simulink model "pfa1008"  (R2025a)
settings: Solver=VariableStepAuto  StartTime=0.0  StopTime=1e-4  RelTol=1e-3
InitFcn:
  | coeffs;
undefined symbols (not defined in the file or in its folder): S, vsva2197, xcvc1902
libraries: aieBasic x20, aieUtilities x5, dspsrcs4 x4, hlsBasic x2, vmcUtilities x1
(part 1 of 2)
settings Model: Creator=robg  LastModifiedBy=sdegala
settings RTWCC: GPUComputeCapability=3.5

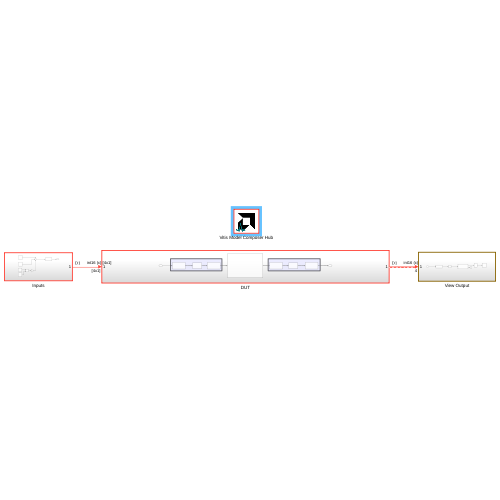
[thumbnail: Simulink's stored preview of the top-level diagram]
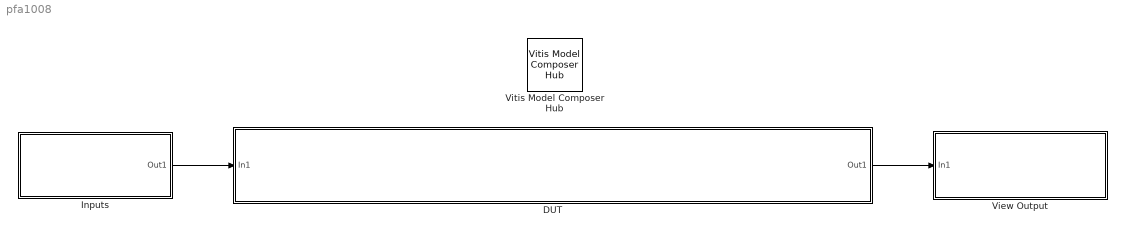
== system pfa1008 ==
  DUT : Subsystem
  Inputs : Subsystem
  View Output : Subsystem
  Vitis Model Composer Hub : vmcUtilities/Vitis Model Composer Hub  Tag=genX  CodeGeneration=off  SubsystemName=DUT  DUTSubsystemName=pfa1008  BlockHierPath=pfa1008/DUT  CompilationType=VitisCompilation  SubsystemType=DUTNode  ExportTypeV2=Graph Code  AIEArrayConfig=Use entire AIE array  StartColumn=1  NumberOfColumns=1  TargetDirectory=./code  exportDesign=on  analyzeDesign=off  validateDesignOnHw=off  ExportType=Vitis Subsystem  IpVendor=xilinx.com  IpLibrary=hls  IpName=pfa1008_permute_o_wrapper  IpVersion=1.0  IpHWLanguage=Verilog  AieCompilerOptions={}  AieSimulatorOptions={''}  CreateTestbench=off  TestbenchStackSize=10  RunRtlSim=off  RunCSim=off  RunAieSim=on  AieSimTimeout=50000  RunAieSimProfiling=off  LaunchVitisAnalyzer=off  PlotOutput=off  RunX86Sim=off  X86SimTimeout=10  GenHwImage=off  GenLibadfXo=on  GenHwValidationCode=on  PlatformType=Specify Platform  Platform=/proj/xbuilds/SWIP/9999.0_0818_1732/installs/lin64/2025.2/Vitis/base_platforms/xilinx_vck190_base_202520_1/xilinx_vck190_base_202520_1.xpfm  HwSystemType=Baremetal  HwValidationTarget=hw_emu  ProjDevice=Versal VCK190 Evaluation Platform (xcvc1902-vsva2197-2MP-e-S)  ProjDevicePart=xcvc1902-vsva2197-2MP-e-S  AIEType=AIE  SamplePeriod=-1  ClockFrequency=200  DataPathParallelism=1  xilinxfamily=versalaicore  part=xcvc1902  speed=-2MP-e-S  package=vsva2197  directory=./netlist  testbench=off  incr_netlist=off  synthesis_tool=Vivado  clock_wrapper=Clock Enables  dbl_ovrd=According to Block Masks  dcm_input_clock_period=10  sysclk_period=10  simulink_period=1  eval_field=0  IPInfoJsonString="{\"DUTSubsystemName\":\"DUT\",\"HLSKernel\":[{\"SubsystemName\":\"pfa1008_permute_i_wrapper\",\"FpgaClockFreq\":\"200\",\"IPName\":\"pfa1008_permute_i_wrapper\",\"IPLibrary\":\"hls\",\"TargetDirectory\":\"./code\",\"FreqHz\":\"200000000\",\"KernelFunction\":\"pfa1008_permute_i_wrapper\"},{\"SubsystemName\":\"pfa1008_permute_o_wrapper\",\"FpgaClockFreq\":\"200\",\"IPName\":\"pfa1008_permute_o_wrapper\",\"IPLibrary\":\"hls\",\"TargetDirectory\":\"./code\",\"FreqHz\":\"200000000\",\"KernelFunction\":\"pfa1008_permute_o_wrapper\"}],\"SubsystemTag\":\"DUTNode\",\"AIESubsystem\":{\"SubsystemName\":\"pfa1008_aie\",\"TargetDirectory\":\"./code\",\"AIEArrayConfig\":\"Use entire AIE array\",\"StartColumn\":\"1\",\"NumberOfColumns\":\"1\"}}"  LogFileName=/proj/xhdhdstaff5/sdegala/Head1/HEAD/VMC_2025_2_July/Examples/AIENGINE_plus_PL/AIE_HLS/Prime_Factor_FFT/code/model_composer.log  NThreads=4  IPConfigFile=/tmp/vmctmp-6835010160091439353/pfa1008_ipconfig.json
  wires:
  Inputs/1(Out1) -> DUT/1(In1)
  DUT/1(Out1) -> View Output/1(In1)

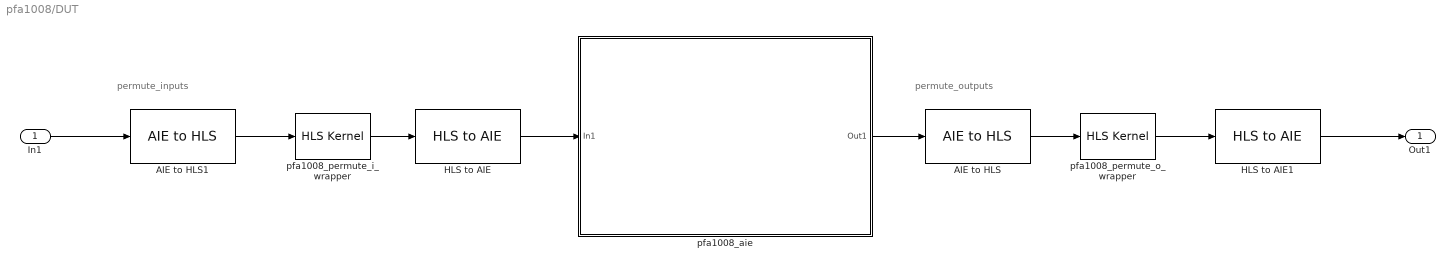
== system pfa1008/DUT ==
  note: permute_outputs
  note: permute_inputs
  In1 : Inport
  AIE to HLS : aieUtilities/AIE to HLS  OutputType=ufix128  OutputSize=252  AllowMultiRate=off  InputType=int8
  AIE to HLS1 : aieUtilities/AIE to HLS  OutputType=ufix128  OutputSize=1  AllowMultiRate=off  InputType=int8
  HLS to AIE : aieUtilities/HLS to AIE  OutputType=cint16  OutputSize=1008  AllowMultiRate=off  InputType=cint16
  HLS to AIE1 : aieUtilities/HLS to AIE  OutputType=cint16  OutputSize=4  AllowMultiRate=off  InputType=cint16
  pfa1008_aie : Subsystem
  pfa1008_permute_i_wrapper : hlsBasic/HLS Kernel  PortNames={'return'; 'sig_i'; 'sig_o'}  PortSerializedTypes={'{Bv}'; '{R{Thls::stream{2{t{Tap_uint{1{t{}128}}}}{t{}0}}}}'; '{R{Thls::stream{2{t{Tap_uint{1{t{}128}}}}{t{}0}}}}'}  FunctionTemplateSpecKind=none  FunctionTemplateParamNames={}  FunctionTemplateParamKinds={}  FunctionTemplateParamTypes={}  FunctionTemplateParamValues={}  PortSynchronicities={'auto'; 'auto'}  PortSignalSizes={0.000000000000000000e+00; 2.520000000000000000e+02}  PortParameterValues={}  PortAttributesTable={ 'Input', 'sig_i', 'hls::stream< ap_uint< 128 >, 0 > &', '', ''; 'Output', 'sig_o', 'hls::stream< ap_uint< 128 >, 0 > &', '', '252' }  PortAttributesEnablement={'off', 'off', 'off', 'off', 'off';'off', 'off', 'off', 'off', 'on'}  PortParametersTable={}  SampleTime=-1  PortDirectionTable={ 'sig_i', 'hls::stream< ap_uint< 128 >, 0 > &', 'Input', 'Port'; 'sig_o', 'hls::stream< ap_uint< 128 >, 0 > &', 'Output', 'Port' }  FunctionTemplateParams={}  FunctionTemplateParamsEnables={}  FunctionTemplateParamsVisible=off  FunctionDeclTypeOptions=C[1 1]@t7@<empty>  PortDirectionTabVisible=on  ArgDirections={1.000000000000000000e+00; 2.000000000000000000e+00}  ArgInterfaceTypes={1.000000000000000000e+00; 1.000000000000000000e+00}  FunctionIndex=1  FormalArgDecls={'hls::stream< ap_uint< 128 >, 0 > & sig_i', 'hls::stream< ap_uint< 128 >, 0 > & sig_o'}  SimLibPath=''  FunctionTabVisible=on  FunctionDescription=void pfa1008_permute_i_wrapper(hls::stream< ap_uint< 128 >, 0 > & sig_i, hls::stream< ap_uint< 128 >, 0 > & sig_o)  blockJsonConstraints=[]  deprecateConstraints=0  KernelHeaderFile=./hls/pfa1008_permute_i/pfa1008_permute_i.h  KernelFunction=pfa1008_permute_i_wrapper  KernelFunctionSelect=<empty>  KernelSourceFile=./hls/pfa1008_permute_i/pfa1008_permute_i.cpp  KernelSearchPaths={}  PreProcOptions={}
  pfa1008_permute_o_wrapper : hlsBasic/HLS Kernel  PortNames={'return'; 'sig_i'; 'sig_o'}  PortSerializedTypes={'{Bv}'; '{R{Thls::stream{2{t{Tap_uint{1{t{}128}}}}{t{}0}}}}'; '{R{Thls::stream{2{t{Tap_uint{1{t{}128}}}}{t{}0}}}}'}  FunctionTemplateSpecKind=none  FunctionTemplateParamNames={}  FunctionTemplateParamKinds={}  FunctionTemplateParamTypes={}  FunctionTemplateParamValues={}  PortSynchronicities={'auto'; 'auto'}  PortSignalSizes={0.000000000000000000e+00; 1.000000000000000000e+00}  PortParameterValues={}  PortAttributesTable={ 'Input', 'sig_i', 'hls::stream< ap_uint< 128 >, 0 > &', '', ''; 'Output', 'sig_o', 'hls::stream< ap_uint< 128 >, 0 > &', '', '1' }  PortAttributesEnablement={'off', 'off', 'off', 'off', 'off';'off', 'off', 'off', 'off', 'on'}  PortParametersTable={}  SampleTime=-1  PortDirectionTable={ 'sig_i', 'hls::stream< ap_uint< 128 >, 0 > &', 'Input', 'Port'; 'sig_o', 'hls::stream< ap_uint< 128 >, 0 > &', 'Output', 'Port' }  FunctionTemplateParams={}  FunctionTemplateParamsEnables={}  FunctionTemplateParamsVisible=off  FunctionDeclTypeOptions=C[1 1]@t7@<empty>  PortDirectionTabVisible=on  ArgDirections={1.000000000000000000e+00; 2.000000000000000000e+00}  ArgInterfaceTypes={1.000000000000000000e+00; 1.000000000000000000e+00}  FunctionIndex=1  FormalArgDecls={'hls::stream< ap_uint< 128 >, 0 > & sig_i', 'hls::stream< ap_uint< 128 >, 0 > & sig_o'}  SimLibPath=''  FunctionTabVisible=on  FunctionDescription=void pfa1008_permute_o_wrapper(hls::stream< ap_uint< 128 >, 0 > & sig_i, hls::stream< ap_uint< 128 >, 0 > & sig_o)  blockJsonConstraints=[]  deprecateConstraints=0  KernelHeaderFile=./hls/pfa1008_permute_o/pfa1008_permute_o.h  KernelFunction=pfa1008_permute_o_wrapper  KernelFunctionSelect=<empty>  KernelSourceFile=./hls/pfa1008_permute_o/pfa1008_permute_o.cpp  KernelSearchPaths={}  PreProcOptions={}
  Out1 : Outport
  wires:
  HLS to AIE/1 -> pfa1008_aie/1(In1)
  HLS to AIE1/1 -> Out1/1
  In1/1 -> AIE to HLS1/1
  AIE to HLS1/1 -> pfa1008_permute_i_wrapper/1
  pfa1008_permute_i_wrapper/1 -> HLS to AIE/1
  pfa1008_aie/1(Out1) -> AIE to HLS/1
  pfa1008_permute_o_wrapper/1 -> HLS to AIE1/1
  AIE to HLS/1 -> pfa1008_permute_o_wrapper/1

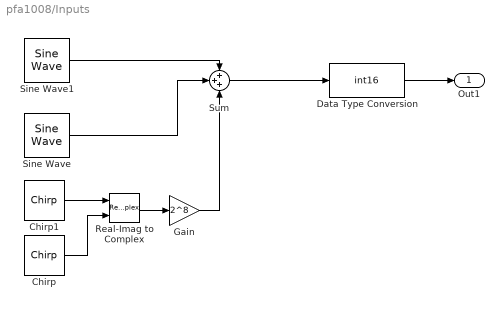
== system pfa1008/Inputs ==
  Chirp : dspsrcs4/Chirp  sweep=Linear  mode=Unidirectional  f0=100/1008*(1e9)  f1=200/1008*(1e9)  t1=4032*(1e-9)  Tsweep=4032*(1e-9)  phase=0  Ts=1e-9  spf=4  datatype=double  OutputFrames=off
  Chirp1 : dspsrcs4/Chirp  sweep=Linear  mode=Unidirectional  f0=100/1008*(1e9)  f1=200/1008*(1e9)  t1=4032*(1e-9)  Tsweep=4032*(1e-9)  phase=pi/2  Ts=1e-9  spf=4  datatype=double  OutputFrames=off
  Data Type Conversion : DataTypeConversion  OutDataTypeStr=int16  SaturateOnIntegerOverflow=off  RndMeth=Floor
  Gain : Gain  Gain=2^8  OutDataTypeStr=double
  Real-Imag to Complex : RealImagToComplex
  Sine Wave : dspsrcs4/Sine Wave  Amplitude=2^8  Frequency=128/1008*(1e9)  Phase=0  SampleMode=Discrete  OutComplex=Complex  CompMethod=Trigonometric fcn  TableSize=Speed  SampleTime=1e-9  SamplesPerFrame=4  ResetState=Restart at time zero  OutputFrames=off  dataType=double  wordLen=16  udDataType=sfix(16)  fracBitsMode=Best precision  numFracBits=15  OutDataTypeStr=double  LastOutDataTypeStr=double
  Sine Wave1 : dspsrcs4/Sine Wave  Amplitude=2^8  Frequency=400/1008*(1e9)  Phase=0  SampleMode=Discrete  OutComplex=Complex  CompMethod=Trigonometric fcn  TableSize=Speed  SampleTime=1e-9  SamplesPerFrame=4  ResetState=Restart at time zero  OutputFrames=off  dataType=double  wordLen=16  udDataType=sfix(16)  fracBitsMode=Best precision  numFracBits=15  OutDataTypeStr=double  LastOutDataTypeStr=double
  Sum : Sum  Inputs=+++
  Out1 : Outport
  wires:
  Sine Wave1/1 -> Sum/1
  Sine Wave/1 -> Sum/2
  Sum/1 -> Data Type Conversion/1
  Data Type Conversion/1 -> Out1/1
  Gain/1 -> Sum/3
  Real-Imag to Complex/1 -> Gain/1
  Chirp/1 -> Real-Imag to Complex/2
  Chirp1/1 -> Real-Imag to Complex/1

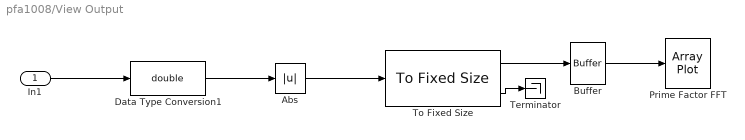
== system pfa1008/View Output ==
  In1 : Inport
  Abs : Abs  OutDataTypeStr=double  SaturateOnIntegerOverflow=off
  Buffer : Buffer  N=1008  OutputFrames=off
  Data Type Conversion1 : DataTypeConversion  OutDataTypeStr=double  SaturateOnIntegerOverflow=off  RndMeth=Floor
  Prime Factor FFT : ArrayPlot  WindowPosition=[1116.000000,386.000000,800.000000,500.000000,]  Visible=on  ScopeFrameLocation=window  MaximizeAxes=Off  YLimits=[-4095.8765 36862.8885]
  Terminator : Terminator
  To Fixed Size : aieUtilities/To Fixed Size  Mode=Produce a valid output signal  OutputSize=Inherit: Same as input  CopyMethod=Buffer samples to form output  HasStatusOutput=on
  wires:
  Abs/1 -> To Fixed Size/1
  Data Type Conversion1/1 -> Abs/1
  To Fixed Size/2 -> Terminator/1
  Buffer/1 -> Prime Factor FFT/1
  To Fixed Size/1 -> Buffer/1
  In1/1 -> Data Type Conversion1/1

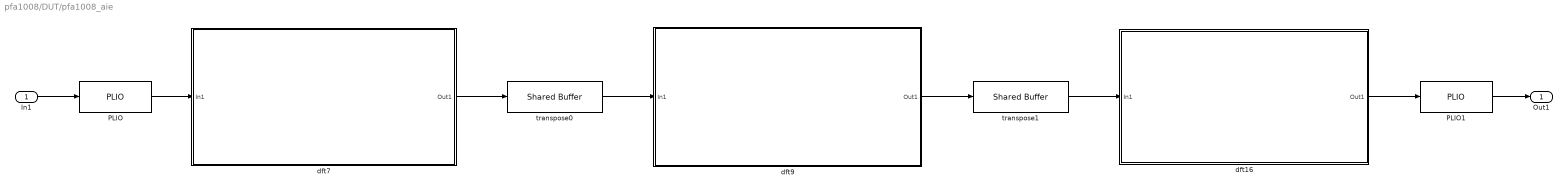
== system pfa1008/DUT/pfa1008_aie ==
  In1 : Inport
  PLIO : aieBasic/PLIO  PlioWidth=64  PlioFreqSpec=on  PlioFreq=625  ColLocation=0  channel=0  blockJsonConstraints=[]  deprecateConstraints=0
  PLIO1 : aieBasic/PLIO  PlioWidth=64  PlioFreqSpec=on  PlioFreq=625  ColLocation=0  channel=0  blockJsonConstraints=[]  deprecateConstraints=0
  dft16 : Subsystem
  dft7 : Subsystem
  dft9 : Subsystem
  transpose0 : aieBasic/Shared Buffer  DataType=cint16  NumBuffer=2  BufferDim=[8,16,16]  NumInput=1  NumOutput=1  RepetitionCount=0  Input0Tiling=struct('buffer_dimension', [8,16,16], 'tiling_dimension', [1,1,1], 'offset', [0,0,0], 'tile_traversal', [struct('dimension', 0, 'stride', 1, 'wrap', 7) struct('dimension', 1, 'stride', 1, 'wrap', 9) struct('dimension', 2, 'stride', 1, 'wrap', 16)])  Input1Tiling=[]  Input2Tiling=[]  Input3Tiling=[]  Input4Tiling=[]  Input5Tiling=[]  Output0Tiling=struct('buffer_dimension', [8,16,16], 'tiling_dimension', [1,1,1], 'offset', [0,0,0], 'tile_traversal', [struct('dimension', 1, 'stride', 1, 'wrap', 9) struct('dimension', 2, 'stride', 1, 'wrap', 16) struct('dimension', 0, 'stride', 1, 'wrap', 7)])  Output1Tiling=[]  Output2Tiling=[]  Output3Tiling=[]  Output4Tiling=[]  Output5Tiling=[]  InBuffDims={8, 16, 16}  InTilingDims={1, 1, 1}  InOffsets={0, 0, 0}  InTileTraveseDims={0,1,2}  InTileTraveseStrides={1,1,1}  InTileTraveseWraps={7,9,16}  InPacketPortIDs={}  InRepetitions={}  InBoundaryDims={}  OutBuffDims={8, 16, 16}  OutTilingDims={1, 1, 1}  OutOffsets={0, 0, 0}  OutTileTraveseDims={1,2,0}  OutTileTraveseStrides={1,1,1}  OutTileTraveseWraps={9,16,7}  OutPacketPortIDs={}  OutRepetitions={}  OutBoundaryDims={}  BufferDimStr={8, 16, 16}  blockJsonConstraints=[]  deprecateConstraints=0
  transpose1 : aieBasic/Shared Buffer  DataType=cint16  NumBuffer=2  BufferDim=[8,16,16]  NumInput=1  NumOutput=1  RepetitionCount=0  Input0Tiling=struct('buffer_dimension', [8,16,16], 'tiling_dimension', [1,1,1], 'offset', [0,0,0], 'tile_traversal', [struct('dimension', 1, 'stride', 1, 'wrap', 9) struct('dimension', 2, 'stride', 1, 'wrap', 16) struct('dimension', 0, 'stride', 1, 'wrap', 7)])  Input1Tiling=[]  Input2Tiling=[]  Input3Tiling=[]  Input4Tiling=[]  Input5Tiling=[]  Output0Tiling=struct('buffer_dimension', [8,16,16], 'tiling_dimension', [1,1,1], 'offset', [0,0,0], 'tile_traversal', [struct('dimension', 2, 'stride', 1, 'wrap', 16) struct('dimension', 1, 'stride', 1, 'wrap', 9) struct('dimension', 0, 'stride', 1, 'wrap', 7)])  Output1Tiling=[]  Output2Tiling=[]  Output3Tiling=[]  Output4Tiling=[]  Output5Tiling=[]  InBuffDims={8, 16, 16}  InTilingDims={1, 1, 1}  InOffsets={0, 0, 0}  InTileTraveseDims={1,2,0}  InTileTraveseStrides={1,1,1}  InTileTraveseWraps={9,16,7}  InPacketPortIDs={}  InRepetitions={}  InBoundaryDims={}  OutBuffDims={8, 16, 16}  OutTilingDims={1, 1, 1}  OutOffsets={0, 0, 0}  OutTileTraveseDims={2,1,0}  OutTileTraveseStrides={1,1,1}  OutTileTraveseWraps={16,9,7}  OutPacketPortIDs={}  OutRepetitions={}  OutBoundaryDims={}  BufferDimStr={8, 16, 16}  blockJsonConstraints=[]  deprecateConstraints=0
  Out1 : Outport
  wires:
  PLIO1/1 -> Out1/1
  In1/1 -> PLIO/1
  PLIO/1 -> dft7/1(In1)
  dft7/1(Out1) -> transpose0/1
  transpose0/1 -> dft9/1(In1)
  dft9/1(Out1) -> transpose1/1
  transpose1/1 -> dft16/1(In1)
  dft16/1(Out1) -> PLIO1/1

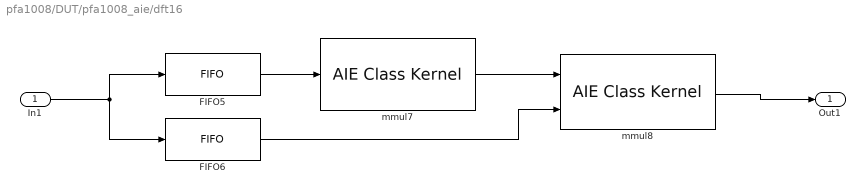
== system pfa1008/DUT/pfa1008_aie/dft16 ==
  In1 : Inport
  FIFO5 : aieBasic/FIFO  FifoDepth=32  FIFOType=0  TileType=0  RowLocation=0  ColLocation=0  channel=0  blockJsonConstraints=[]  deprecateConstraints=0
  FIFO6 : aieBasic/FIFO  FifoDepth=32  FIFOType=0  TileType=0  RowLocation=0  ColLocation=0  channel=0  blockJsonConstraints=[]  deprecateConstraints=0
  mmul7 : aieBasic/AIE Class Kernel  KernelAllAttrs=|  PortNames={'sig_i'; 'acc_o'}  PortSerializedTypes={'{Q2{R{Tadf::input_buffer{2{t{Scint16}}{t{Tadf::extents{1{t{}1008}}}}}}}}'; '{Q2{P{Toutput_cascade{2{t{Scacc64}}{t{Bv}}}}}}'}  PortWindowSizes={1.008000000000000000e+03; 0.000000000000000000e+00}  PortWindowMargins={0.000000000000000000e+00; 0.000000000000000000e+00}  PortSynchronicities={'sync', 'auto'}  PortSignalSizes={0.000000000000000000e+00; 1.008000000000000000e+03}  ClassTemplateSpecKind=none  ClassTemplateParamNames={}  ClassTemplateParamKinds={}  ClassTemplateParamTypes={}  ClassTemplateParamValues={}  ClassCtorParamNames={'coeff_i'}  ClassCtorParamSerializedTypes={'{R{C{Scint16}256}}'}  ClassCtorParamValues={'[32767;32767;32767;32767;32767;32767;32767;32767;32767;30274-12540i;23170-23170i;12540-30274i;0-32768i;-12540-30274i;-23170-23170i;-30274-12540i;32767;23170-23170i;0-32768i;-23170-23170i;-32768;-23170+23170i;0+32767i;23170+23170i;32767;12540-30274i;-23170-23170i;-30274+12540i;0+32767i;30274+12540i;23170-23170i;-12540-30274i;32767;0-32768i;-32768;0+32767i;32767;0-32768i;-32768;0+32767i;32767;-12540-30274i;-23170+23170i;30274+12540i;0-32768i;-30274+12540i;23170+23170i;12540-30274i;32767;-23170-23170i;0+32767i;23170-23170i;-32768;23170+23170i;0-32768i;-23170+23170i;32767;-30274-12540i;23170+23170i;-12540-30274i;0+32767i;12540-30274i;-23170+23170i;30274-12540i;32767;-32768;32767;-32768;32767;-32768;32767;-32768;32767;-30274+12540i;23170-23170i;-12540+30274i;0-32768i;12540+30274i;-23170-23170i;30274+12540i;32767;-23170+23170i;0-32768i;23170+23170i;-32768;23170-23170i;0+32767i;-23170-23170i;32767;-12540+30274i;-23170-23170i;30274-12540i;0+32767i;-30274-12540i;23170-23170i;12540+30274i;32767;0+32767i;-32768;0-32768i;32767;0+32767i;-32768;0-32768i;32767;12540+30274i;-23170+23170i;-30274-12540i;0-32768i;30274-12540i;23170+23170i;-12540+30274i;32767;23170+23170i;0+32767i;-23170+23170i;-32768;-23170-23170i;0-32768i;23170-23170i;32767;30274+12540i;23170+23170i;12540+30274i;0+32767i;-12540+30274i;-23170+23170i;-30274+12540i;32767;32767;32767;32767;32767;32767;32767;32767;-32768;-30274+12540i;-23170+23170i;-12540+30274i;0+32767i;12540+30274i;23170+23170i;30274+12540i;32767;23170-23170i;0-32768i;-23170-23170i;-32768;-23170+23170i;0+32767i;23170+23170i;-32768;-12540+30274i;23170+23170i;30274-12540i;0-32768i;-30274-12540i;-23170+23170i;12540+30274i;32767;0-32768i;-32768;0+32767i;32767;0-32768i;-32768;0+32767i;-32768;12540+30274i;23170-23170i;-30274-12540i;0+32767i;30274-12540i;-23170-23170i;-12540+30274i;32767;-23170-23170i;0+32767i;23170-23170i;-32768;23170+23170i;0-32768i;-23170+23170i;-32768;30274+12540i;-23170-23170i;12540+30274i;0-32768i;-12540+30274i;23170-23170i;-30274+12540i;32767;-32768;32767;-32768;32767;-32768;32767;-32768;-32768;30274-12540i;-23170+23170i;12540-30274i;0+32767i;-12540-30274i;23170+23170i;-30274-12540i;32767;-23170+23170i;0-32768i;23170+23170i;-32768;23170-23170i;0+32767i;-23170-23170i;-32768;12540-30274i;23170+23170i;-30274+12540i;0-32768i;30274+12540i;-23170+23170i;-12540-30274i;32767;0+32767i;-32768;0-32768i;32767;0+32767i;-32768;0-32768i;-32768;-12540-30274i;23170-23170i;30274+12540i;0+32767i;-30274+12540i;-23170-23170i;12540-30274i;32767;23170+23170i;0+32767i;-23170+23170i;-32768;-23170-23170i;0-32768i;23170-23170i;-32768;-30274-12540i;-23170-23170i;-12540-30274i;0-32768i;12540-30274i;23170-23170i;30274-12540i]'}  ClassIndex=1  ClassCtorIndex=1  ClassTabVisible=on  ClassTemplateParamsVisible=off  ClassCtorDeclVisible=on  ClassCtorParamsVisible=on  FunctionTabVisible=on  FunctionDecl=|  PortAttrs={ 'input', 'sig_i', 'adf::input_buffer< cint16, adf::extents< 1008 > > & restrict', '1008', '0', 'sync', ''; 'output', 'acc_o', 'output_cascade< cacc64, void > * restrict', '', '', '', '1008' }  PortAttrsEnables={'off', 'off', 'off', 'off', 'off', 'off', 'off';'off', 'off', 'off', 'off', 'off', 'off', 'on'}  SampleTime=-1  ClassDeclTypeOptions=C[1 1]@t14@class dft16_0;  ClassDecl=class dft16_0;  ClassTemplateParams={}  ClassTemplateParamsEnables={}  ClassCtorDeclTypeOptions=C[1 1]@t37@dft16_0(cint16 ( & coeff_i ) [ 256 ])  ClassCtorDecl=dft16_0(cint16 ( & coeff_i ) [ 256 ])  ClassCtorParams={ 'coeff_i', 'cint16 ( &) [ 256 ]', 'DFT16_TWID' }  KernelHeaderFile=dft16_mmul0.h  KernelClassName=dft16_0  KernelFunction=run  KernelSourceFile=dft16_mmul0.cpp  KernelSearchPaths={'./aie/dft16'}  PreProcOptions={}  blockJsonConstraints="{\"type\":\"constraint\",\"constraintType\":\"location_kernel\",\"sid\":\"56\",\"lhs\":{\"type\":\"location\",\"templParam\":\"kernel\",\"args\":{\"type\":\"kernel\",\"name\":\"pfa1008/pfa1008_dut/pfa1008_aie/dft16/mmul7\",\"sid\":\"56\"}},\"rhs\":{\"type\":\"tile\",\"args\":[{\"type\":\"evaluable\",\"expr\":\"21\",\"value\":21},{\"type\":\"evaluable\",\"expr\":\"0\",\"value\":0}]},\"equality\":true}"
      KernelAllAttrs=|
      | s[12;12;9;9;19;14;21;23;21;23;24;21;15;17;12;24;26;26;26;27;28;9;21;23;23;23;24;25;14;19;19;29]@FunctionNameDeclFileNamePortNamesPortTypesPortSerializedTypesPortDirectionsPortWindowSizeEnablesPortWindowMarginEnablesPortBufferSizeEnablesPortBufferMarginEnablesPortSynchronicityEnablesPortSignalSizeEnablesPortBufferSizesPortBufferMarginsFunctionDeclFunctionTemplateSpecKindFunctionTemplateParamNamesFunctionTemplateParamKindsFunctionTemplateParamTypesFunctionTemplateParamValuesFunctionTemplateParamEnablesClassDeclClassTemplateSpecKindClassTemplateParamNamesClassTemplateParamKindsClassTemplateParamTypesClassTemplateParamValuesClassTemplateParamEnablesClassCtorDeclsClassCtorParamNamesClassCtorParamTypesClassCtorParamSerializedTypes[1 1]@C[32 1]@t3@runt28@../../../dft16/dft16_mmul0.hC[2 1]@t5@sig_it5@acc_oC[2 1]@t60@adf::input_buffer< cint16, adf::extents< 1008 > > & restrictt41@output_cascade< cacc64, void > * restrictC[2 1]@t72@{Q2{R{Tadf::input_buffer{2{t{Scint16}}{t{Tadf::extents{1{t{}1008}}}}}}}}t46@{Q2{P{Toutput_cascade{2{t{Scacc64}}{t{Bv}}}}}}C[2 1]@t5@inputt6@outputC[2 1]@l1@l0@C[2 1]@l1@l0@C[2 1]@l1@l0@C[2 1]@l0@l0@C[2 1]@l1@l0@C[2 1]@l0@l1@C[2 1]@t4@1008nC[2 1]@nnt135@void dft16_0::
      | run(adf::input_buffer< cint16, adf::extents< 1008 > > & restrict sig_i, output_cascade< cacc64, void > * restrict acc_o)t4@nonee[0 1]@e[0 1]@e[0 1]@e[0 1]@e[0 1]@t14@class dft16_0;t4@nonee[0 1]@e[0 1]@e[0 1]@e[0 1]@e[0 1]@C[1 1]@t37@dft16_0(cint16 ( & coeff_i ) [ 256 ])C[1 1]@C[1 1]@t7@coeff_iC[1 1]@C[1 1]@t19@cint16 ( &) [ 256 ]C[1 1]@C[1 1]@t18@{R{C{Scint16}256}}
      FunctionDecl=|
      | void dft16_0::
      | run(adf::input_buffer< cint16, adf::extents< 1008 > > & restrict sig_i, output_cascade< cacc64, void > * restrict acc_o)
  mmul8 : aieBasic/AIE Class Kernel  KernelAllAttrs=|  PortNames={'acc_i'; 'sig_i'; 'sig_o'}  PortSerializedTypes={'{Q2{P{Tinput_cascade{2{t{Scacc64}}{t{Bv}}}}}}'; '{Q2{R{Tadf::input_buffer{2{t{Scint16}}{t{Tadf::extents{1{t{}1008}}}}}}}}'; '{Q2{R{Tadf::output_buffer{2{t{Scint16}}{t{Tadf::extents{1{t{}1008}}}}}}}}'}  PortWindowSizes={0.000000000000000000e+00; 1.008000000000000000e+03; 1.008000000000000000e+03}  PortWindowMargins={0.000000000000000000e+00; 0.000000000000000000e+00; 0.000000000000000000e+00}  PortSynchronicities={'auto', 'sync', 'sync'}  PortSignalSizes={0.000000000000000000e+00; 0.000000000000000000e+00; 0.000000000000000000e+00}  ClassTemplateSpecKind=none  ClassTemplateParamNames={}  ClassTemplateParamKinds={}  ClassTemplateParamTypes={}  ClassTemplateParamValues={}  ClassCtorParamNames={'coeff_i'}  ClassCtorParamSerializedTypes={'{R{C{Scint16}256}}'}  ClassCtorParamValues={'[32767;32767;32767;32767;32767;32767;32767;32767;32767;30274-12540i;23170-23170i;12540-30274i;0-32768i;-12540-30274i;-23170-23170i;-30274-12540i;32767;23170-23170i;0-32768i;-23170-23170i;-32768;-23170+23170i;0+32767i;23170+23170i;32767;12540-30274i;-23170-23170i;-30274+12540i;0+32767i;30274+12540i;23170-23170i;-12540-30274i;32767;0-32768i;-32768;0+32767i;32767;0-32768i;-32768;0+32767i;32767;-12540-30274i;-23170+23170i;30274+12540i;0-32768i;-30274+12540i;23170+23170i;12540-30274i;32767;-23170-23170i;0+32767i;23170-23170i;-32768;23170+23170i;0-32768i;-23170+23170i;32767;-30274-12540i;23170+23170i;-12540-30274i;0+32767i;12540-30274i;-23170+23170i;30274-12540i;32767;-32768;32767;-32768;32767;-32768;32767;-32768;32767;-30274+12540i;23170-23170i;-12540+30274i;0-32768i;12540+30274i;-23170-23170i;30274+12540i;32767;-23170+23170i;0-32768i;23170+23170i;-32768;23170-23170i;0+32767i;-23170-23170i;32767;-12540+30274i;-23170-23170i;30274-12540i;0+32767i;-30274-12540i;23170-23170i;12540+30274i;32767;0+32767i;-32768;0-32768i;32767;0+32767i;-32768;0-32768i;32767;12540+30274i;-23170+23170i;-30274-12540i;0-32768i;30274-12540i;23170+23170i;-12540+30274i;32767;23170+23170i;0+32767i;-23170+23170i;-32768;-23170-23170i;0-32768i;23170-23170i;32767;30274+12540i;23170+23170i;12540+30274i;0+32767i;-12540+30274i;-23170+23170i;-30274+12540i;32767;32767;32767;32767;32767;32767;32767;32767;-32768;-30274+12540i;-23170+23170i;-12540+30274i;0+32767i;12540+30274i;23170+23170i;30274+12540i;32767;23170-23170i;0-32768i;-23170-23170i;-32768;-23170+23170i;0+32767i;23170+23170i;-32768;-12540+30274i;23170+23170i;30274-12540i;0-32768i;-30274-12540i;-23170+23170i;12540+30274i;32767;0-32768i;-32768;0+32767i;32767;0-32768i;-32768;0+32767i;-32768;12540+30274i;23170-23170i;-30274-12540i;0+32767i;30274-12540i;-23170-23170i;-12540+30274i;32767;-23170-23170i;0+32767i;23170-23170i;-32768;23170+23170i;0-32768i;-23170+23170i;-32768;30274+12540i;-23170-23170i;12540+30274i;0-32768i;-12540+30274i;23170-23170i;-30274+12540i;32767;-32768;32767;-32768;32767;-32768;32767;-32768;-32768;30274-12540i;-23170+23170i;12540-30274i;0+32767i;-12540-30274i;23170+23170i;-30274-12540i;32767;-23170+23170i;0-32768i;23170+23170i;-32768;23170-23170i;0+32767i;-23170-23170i;-32768;12540-30274i;23170+23170i;-30274+12540i;0-32768i;30274+12540i;-23170+23170i;-12540-30274i;32767;0+32767i;-32768;0-32768i;32767;0+32767i;-32768;0-32768i;-32768;-12540-30274i;23170-23170i;30274+12540i;0+32767i;-30274+12540i;-23170-23170i;12540-30274i;32767;23170+23170i;0+32767i;-23170+23170i;-32768;-23170-23170i;0-32768i;23170-23170i;-32768;-30274-12540i;-23170-23170i;-12540-30274i;0-32768i;12540-30274i;23170-23170i;30274-12540i]'}  ClassIndex=1  ClassCtorIndex=1  ClassTabVisible=on  ClassTemplateParamsVisible=off  ClassCtorDeclVisible=on  ClassCtorParamsVisible=on  FunctionTabVisible=on  FunctionDecl=|  PortAttrs={ 'input', 'acc_i', 'input_cascade< cacc64, void > * restrict', '', '', '', ''; 'input', 'sig_i', 'adf::input_buffer< cint16, adf::extents< 1008 > > & restrict', '1008', '0', 'sync', ''; 'output', 'sig_o', 'adf::output_buffer< cint16, adf::extents< 1008 > > & restrict', '1008', '', 'sync', '' }  PortAttrsEnables={'off', 'off', 'off', 'off', 'off', 'off', 'off';'off', 'off', 'off', 'off', 'off', 'off', 'off';'off', 'off', 'off', 'off', 'off', 'off', 'off'}  SampleTime=-1  ClassDeclTypeOptions=C[1 1]@t14@class dft16_1;  ClassDecl=class dft16_1;  ClassTemplateParams={}  ClassTemplateParamsEnables={}  ClassCtorDeclTypeOptions=C[1 1]@t37@dft16_1(cint16 ( & coeff_i ) [ 256 ])  ClassCtorDecl=dft16_1(cint16 ( & coeff_i ) [ 256 ])  ClassCtorParams={ 'coeff_i', 'cint16 ( &) [ 256 ]', 'DFT16_TWID' }  KernelHeaderFile=dft16_mmul1.h  KernelClassName=dft16_1  KernelFunction=run  KernelSourceFile=dft16_mmul1.cpp  KernelSearchPaths={'./aie/dft16'}  PreProcOptions={}  blockJsonConstraints="{\"type\":\"constraint\",\"constraintType\":\"location_kernel\",\"sid\":\"57\",\"lhs\":{\"type\":\"location\",\"templParam\":\"kernel\",\"args\":{\"type\":\"kernel\",\"name\":\"pfa1008/pfa1008_dut/pfa1008_aie/dft16/mmul8\",\"sid\":\"57\"}},\"rhs\":{\"type\":\"tile\",\"args\":[{\"type\":\"evaluable\",\"expr\":\"22\",\"value\":22},{\"type\":\"evaluable\",\"expr\":\"0\",\"value\":0}]},\"equality\":true}"
      KernelAllAttrs=|
      | s[12;12;9;9;19;14;21;23;21;23;24;21;15;17;12;24;26;26;26;27;28;9;21;23;23;23;24;25;14;19;19;29]@FunctionNameDeclFileNamePortNamesPortTypesPortSerializedTypesPortDirectionsPortWindowSizeEnablesPortWindowMarginEnablesPortBufferSizeEnablesPortBufferMarginEnablesPortSynchronicityEnablesPortSignalSizeEnablesPortBufferSizesPortBufferMarginsFunctionDeclFunctionTemplateSpecKindFunctionTemplateParamNamesFunctionTemplateParamKindsFunctionTemplateParamTypesFunctionTemplateParamValuesFunctionTemplateParamEnablesClassDeclClassTemplateSpecKindClassTemplateParamNamesClassTemplateParamKindsClassTemplateParamTypesClassTemplateParamValuesClassTemplateParamEnablesClassCtorDeclsClassCtorParamNamesClassCtorParamTypesClassCtorParamSerializedTypes[1 1]@C[32 1]@t3@runt28@../../../dft16/dft16_mmul1.hC[3 1]@t5@acc_it5@sig_it5@sig_oC[3 1]@t40@input_cascade< cacc64, void > * restrictt60@adf::input_buffer< cint16, adf::extents< 1008 > > & restrictt61@adf::output_buffer< cint16, adf::extents< 1008 > > & restrictC[3 1]@t45@{Q2{P{Tinput_cascade{2{t{Scacc64}}{t{Bv}}}}}}t72@{Q2{R{Tadf::input_buffer{2{t{Scint16}}{t{Tadf::extents{1{t{}1008}}}}}}}}t73@{Q2{R{Tadf::output_buffer{2{t{Scint16}}{t{Tadf::extents{1{t{}1008}}}}}}}}C[3 1]@t5@inputt5@inputt6@outputC[3 1]@l0@l1@l1@C[3 1]@l0@l1@l0@C[3 1]@l0@l1@l1@C[3 1]@l0@l0@l0@C[3 1]@l0@l1@l1@C[3 1]@l0@l0@l0@C[3 1]@nt4@1008t4@1008C[3 1]@nnnt203@void dft16_1::
      | run(input_cascade< cacc64, void > * restrict acc_i, adf::input_buffer< cint16, adf::extents< 1008 > > & restrict sig_i, adf::output_buffer< cint16, adf::extents< 1008 > > & restrict sig_o)t4@nonee[0 1]@e[0 1]@e[0 1]@e[0 1]@e[0 1]@t14@class dft16_1;t4@nonee[0 1]@e[0 1]@e[0 1]@e[0 1]@e[0 1]@C[1 1]@t37@dft16_1(cint16 ( & coeff_i ) [ 256 ])C[1 1]@C[1 1]@t7@coeff_iC[1 1]@C[1 1]@t19@cint16 ( &) [ 256 ]C[1 1]@C[1 1]@t18@{R{C{Scint16}256}}
      FunctionDecl=|
      | void dft16_1::
      | run(input_cascade< cacc64, void > * restrict acc_i, adf::input_buffer< cint16, adf::extents< 1008 > > & restrict sig_i, adf::output_buffer< cint16, adf::extents< 1008 > > & restrict sig_o)
  Out1 : Outport
  wires:
  FIFO6/1 -> mmul8/2
  mmul7/1 -> mmul8/1
  FIFO5/1 -> mmul7/1
  mmul8/1 -> Out1/1
  In1/1 -> FIFO6/1, FIFO5/1

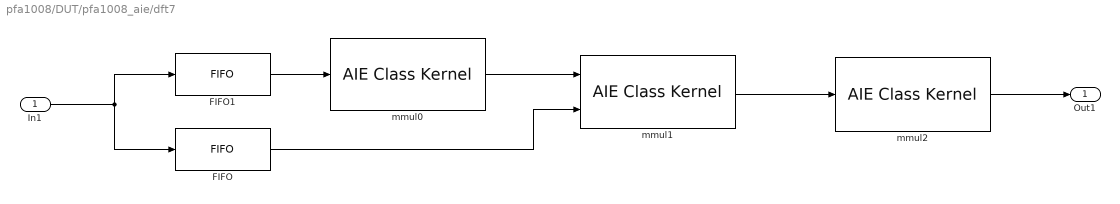
== system pfa1008/DUT/pfa1008_aie/dft7 ==
  In1 : Inport
  FIFO : aieBasic/FIFO  FifoDepth=32  FIFOType=0  TileType=0  RowLocation=0  ColLocation=0  channel=0  blockJsonConstraints=[]  deprecateConstraints=0
  FIFO1 : aieBasic/FIFO  FifoDepth=32  FIFOType=0  TileType=0  RowLocation=0  ColLocation=0  channel=0  blockJsonConstraints=[]  deprecateConstraints=0
  mmul0 : aieBasic/AIE Class Kernel  KernelAllAttrs=|  PortNames={'sig_i'; 'acc_o'}  PortSerializedTypes={'{Q2{R{Tadf::input_buffer{2{t{Scint16}}{t{Tadf::extents{1{t{}1008}}}}}}}}'; '{Q2{P{Toutput_cascade{2{t{Scacc64}}{t{Bv}}}}}}'}  PortWindowSizes={1.008000000000000000e+03; 0.000000000000000000e+00}  PortWindowMargins={0.000000000000000000e+00; 0.000000000000000000e+00}  PortSynchronicities={'sync', 'auto'}  PortSignalSizes={0.000000000000000000e+00; 1.152000000000000000e+03}  ClassTemplateSpecKind=none  ClassTemplateParamNames={}  ClassTemplateParamKinds={}  ClassTemplateParamTypes={}  ClassTemplateParamValues={}  ClassCtorParamNames={'coeff_i'}  ClassCtorParamSerializedTypes={'{R{C{Scint16}32}}'}  ClassCtorParamValues={'[32767;32767;32767;32767;32767;32767;32767;0;32767;20431-25619i;-7292-31946i;-29523-14218i;-29523+14218i;-7292+31946i;20431+25619i;0;32767;-7292-31946i;-29523+14218i;20431+25619i;20431-25619i;-29523-14218i;-7292+31946i;0;32767;-29523-14218i;20431+25619i;-7292-31946i;-7292+31946i;20431-25619i;-29523+14218i;0]'}  ClassIndex=1  ClassCtorIndex=1  ClassTabVisible=on  ClassTemplateParamsVisible=off  ClassCtorDeclVisible=on  ClassCtorParamsVisible=on  FunctionTabVisible=on  FunctionDecl=|  PortAttrs={ 'input', 'sig_i', 'adf::input_buffer< cint16, adf::extents< 1008 > > & restrict', '1008', '0', 'sync', ''; 'output', 'acc_o', 'output_cascade< cacc64, void > * restrict', '', '', '', '1152' }  PortAttrsEnables={'off', 'off', 'off', 'off', 'off', 'off', 'off';'off', 'off', 'off', 'off', 'off', 'off', 'on'}  SampleTime=-1  ClassDeclTypeOptions=C[1 1]@t13@class dft7_0;  ClassDecl=class dft7_0;  ClassTemplateParams={}  ClassTemplateParamsEnables={}  ClassCtorDeclTypeOptions=C[1 1]@t35@dft7_0(cint16 ( & coeff_i ) [ 32 ])  ClassCtorDecl=dft7_0(cint16 ( & coeff_i ) [ 32 ])  ClassCtorParams={ 'coeff_i', 'cint16 ( &) [ 32 ]', 'DFT7_TWID0' }  KernelHeaderFile=dft7_mmul0.h  KernelClassName=dft7_0  KernelFunction=run  KernelSourceFile=dft7_mmul0.cpp  KernelSearchPaths={'./aie/dft7'}  PreProcOptions={}  blockJsonConstraints="{\"type\":\"constraint\",\"constraintType\":\"location_kernel\",\"sid\":\"34\",\"lhs\":{\"type\":\"location\",\"templParam\":\"kernel\",\"args\":{\"type\":\"kernel\",\"name\":\"pfa1008/pfa1008_dut/pfa1008_aie/dft7/mmul0\",\"sid\":\"34\"}},\"rhs\":{\"type\":\"tile\",\"args\":[{\"type\":\"evaluable\",\"expr\":\"18\",\"value\":18},{\"type\":\"evaluable\",\"expr\":\"0\",\"value\":0}]},\"equality\":true}"
      KernelAllAttrs=|
      | s[12;12;9;9;19;14;21;23;21;23;24;21;15;17;12;24;26;26;26;27;28;9;21;23;23;23;24;25;14;19;19;29]@FunctionNameDeclFileNamePortNamesPortTypesPortSerializedTypesPortDirectionsPortWindowSizeEnablesPortWindowMarginEnablesPortBufferSizeEnablesPortBufferMarginEnablesPortSynchronicityEnablesPortSignalSizeEnablesPortBufferSizesPortBufferMarginsFunctionDeclFunctionTemplateSpecKindFunctionTemplateParamNamesFunctionTemplateParamKindsFunctionTemplateParamTypesFunctionTemplateParamValuesFunctionTemplateParamEnablesClassDeclClassTemplateSpecKindClassTemplateParamNamesClassTemplateParamKindsClassTemplateParamTypesClassTemplateParamValuesClassTemplateParamEnablesClassCtorDeclsClassCtorParamNamesClassCtorParamTypesClassCtorParamSerializedTypes[1 1]@C[32 1]@t3@runt26@../../../dft7/dft7_mmul0.hC[2 1]@t5@sig_it5@acc_oC[2 1]@t60@adf::input_buffer< cint16, adf::extents< 1008 > > & restrictt41@output_cascade< cacc64, void > * restrictC[2 1]@t72@{Q2{R{Tadf::input_buffer{2{t{Scint16}}{t{Tadf::extents{1{t{}1008}}}}}}}}t46@{Q2{P{Toutput_cascade{2{t{Scacc64}}{t{Bv}}}}}}C[2 1]@t5@inputt6@outputC[2 1]@l1@l0@C[2 1]@l1@l0@C[2 1]@l1@l0@C[2 1]@l0@l0@C[2 1]@l1@l0@C[2 1]@l0@l1@C[2 1]@t4@1008nC[2 1]@nnt134@void dft7_0::
      | run(adf::input_buffer< cint16, adf::extents< 1008 > > & restrict sig_i, output_cascade< cacc64, void > * restrict acc_o)t4@nonee[0 1]@e[0 1]@e[0 1]@e[0 1]@e[0 1]@t13@class dft7_0;t4@nonee[0 1]@e[0 1]@e[0 1]@e[0 1]@e[0 1]@C[1 1]@t35@dft7_0(cint16 ( & coeff_i ) [ 32 ])C[1 1]@C[1 1]@t7@coeff_iC[1 1]@C[1 1]@t18@cint16 ( &) [ 32 ]C[1 1]@C[1 1]@t17@{R{C{Scint16}32}}
      FunctionDecl=|
      | void dft7_0::
      | run(adf::input_buffer< cint16, adf::extents< 1008 > > & restrict sig_i, output_cascade< cacc64, void > * restrict acc_o)
  mmul1 : aieBasic/AIE Class Kernel  KernelAllAttrs=|  PortNames={'acc_i'; 'sig_i'; 'acc_o'}  PortSerializedTypes={'{Q2{P{Tinput_cascade{2{t{Scacc64}}{t{Bv}}}}}}'; '{Q2{R{Tadf::input_buffer{2{t{Scint16}}{t{Tadf::extents{1{t{}1008}}}}}}}}'; '{Q2{P{Toutput_cascade{2{t{Scacc64}}{t{Bv}}}}}}'}  PortWindowSizes={0.000000000000000000e+00; 1.008000000000000000e+03; 0.000000000000000000e+00}  PortWindowMargins={0.000000000000000000e+00; 0.000000000000000000e+00; 0.000000000000000000e+00}  PortSynchronicities={'auto', 'sync', 'auto'}  PortSignalSizes={0.000000000000000000e+00; 0.000000000000000000e+00; 1.152000000000000000e+03}  ClassTemplateSpecKind=none  ClassTemplateParamNames={}  ClassTemplateParamKinds={}  ClassTemplateParamTypes={}  ClassTemplateParamValues={}  ClassCtorParamNames={'coeff_i'}  ClassCtorParamSerializedTypes={'{R{C{Scint16}32}}'}  ClassCtorParamValues={'[32767;-29523+14218i;20431-25619i;-7292+31946i;-7292-31946i;20431+25619i;-29523-14218i;0;32767;-7292+31946i;-29523-14218i;20431-25619i;20431+25619i;-29523+14218i;-7292-31946i;0;32767;20431+25619i;-7292+31946i;-29523+14218i;-29523-14218i;-7292-31946i;20431-25619i;0;0;0;0;0;0;0;0;0]'}  ClassIndex=1  ClassCtorIndex=1  ClassTabVisible=on  ClassTemplateParamsVisible=off  ClassCtorDeclVisible=on  ClassCtorParamsVisible=on  FunctionTabVisible=on  FunctionDecl=|  PortAttrs={ 'input', 'acc_i', 'input_cascade< cacc64, void > * restrict', '', '', '', ''; 'input', 'sig_i', 'adf::input_buffer< cint16, adf::extents< 1008 > > & restrict', '1008', '0', 'sync', ''; 'output', 'acc_o', 'output_cascade< cacc64, void > * restrict', '', '', '', '1152' }  PortAttrsEnables={'off', 'off', 'off', 'off', 'off', 'off', 'off';'off', 'off', 'off', 'off', 'off', 'off', 'off';'off', 'off', 'off', 'off', 'off', 'off', 'on'}  SampleTime=-1  ClassDeclTypeOptions=C[1 1]@t13@class dft7_1;  ClassDecl=class dft7_1;  ClassTemplateParams={}  ClassTemplateParamsEnables={}  ClassCtorDeclTypeOptions=C[1 1]@t35@dft7_1(cint16 ( & coeff_i ) [ 32 ])  ClassCtorDecl=dft7_1(cint16 ( & coeff_i ) [ 32 ])  ClassCtorParams={ 'coeff_i', 'cint16 ( &) [ 32 ]', 'DFT7_TWID1' }  KernelHeaderFile=dft7_mmul1.h  KernelClassName=dft7_1  KernelFunction=run  KernelSourceFile=dft7_mmul1.cpp  KernelSearchPaths={'./aie/dft7'}  PreProcOptions={}  blockJsonConstraints="{\"type\":\"constraint\",\"constraintType\":\"location_kernel\",\"sid\":\"35\",\"lhs\":{\"type\":\"location\",\"templParam\":\"kernel\",\"args\":{\"type\":\"kernel\",\"name\":\"pfa1008/pfa1008_dut/pfa1008_aie/dft7/mmul1\",\"sid\":\"35\"}},\"rhs\":{\"type\":\"tile\",\"args\":[{\"type\":\"evaluable\",\"expr\":\"19\",\"value\":19},{\"type\":\"evaluable\",\"expr\":\"0\",\"value\":0}]},\"equality\":true}"
      KernelAllAttrs=|
      | s[12;12;9;9;19;14;21;23;21;23;24;21;15;17;12;24;26;26;26;27;28;9;21;23;23;23;24;25;14;19;19;29]@FunctionNameDeclFileNamePortNamesPortTypesPortSerializedTypesPortDirectionsPortWindowSizeEnablesPortWindowMarginEnablesPortBufferSizeEnablesPortBufferMarginEnablesPortSynchronicityEnablesPortSignalSizeEnablesPortBufferSizesPortBufferMarginsFunctionDeclFunctionTemplateSpecKindFunctionTemplateParamNamesFunctionTemplateParamKindsFunctionTemplateParamTypesFunctionTemplateParamValuesFunctionTemplateParamEnablesClassDeclClassTemplateSpecKindClassTemplateParamNamesClassTemplateParamKindsClassTemplateParamTypesClassTemplateParamValuesClassTemplateParamEnablesClassCtorDeclsClassCtorParamNamesClassCtorParamTypesClassCtorParamSerializedTypes[1 1]@C[32 1]@t3@runt26@../../../dft7/dft7_mmul1.hC[3 1]@t5@acc_it5@sig_it5@acc_oC[3 1]@t40@input_cascade< cacc64, void > * restrictt60@adf::input_buffer< cint16, adf::extents< 1008 > > & restrictt41@output_cascade< cacc64, void > * restrictC[3 1]@t45@{Q2{P{Tinput_cascade{2{t{Scacc64}}{t{Bv}}}}}}t72@{Q2{R{Tadf::input_buffer{2{t{Scint16}}{t{Tadf::extents{1{t{}1008}}}}}}}}t46@{Q2{P{Toutput_cascade{2{t{Scacc64}}{t{Bv}}}}}}C[3 1]@t5@inputt5@inputt6@outputC[3 1]@l0@l1@l0@C[3 1]@l0@l1@l0@C[3 1]@l0@l1@l0@C[3 1]@l0@l0@l0@C[3 1]@l0@l1@l0@C[3 1]@l0@l0@l1@C[3 1]@nt4@1008nC[3 1]@nnnt182@void dft7_1::
      | run(input_cascade< cacc64, void > * restrict acc_i, adf::input_buffer< cint16, adf::extents< 1008 > > & restrict sig_i, output_cascade< cacc64, void > * restrict acc_o)t4@nonee[0 1]@e[0 1]@e[0 1]@e[0 1]@e[0 1]@t13@class dft7_1;t4@nonee[0 1]@e[0 1]@e[0 1]@e[0 1]@e[0 1]@C[1 1]@t35@dft7_1(cint16 ( & coeff_i ) [ 32 ])C[1 1]@C[1 1]@t7@coeff_iC[1 1]@C[1 1]@t18@cint16 ( &) [ 32 ]C[1 1]@C[1 1]@t17@{R{C{Scint16}32}}
      FunctionDecl=|
      | void dft7_1::
      | run(input_cascade< cacc64, void > * restrict acc_i, adf::input_buffer< cint16, adf::extents< 1008 > > & restrict sig_i, output_cascade< cacc64, void > * restrict acc_o)
  mmul2 : aieBasic/AIE Class Kernel  KernelAllAttrs=|  PortNames={'acc_i'; 'sig_o'}  PortSerializedTypes={'{Q2{P{Tinput_cascade{2{t{Scacc64}}{t{Bv}}}}}}'; '{Q2{R{Tadf::output_buffer{2{t{Scint16}}{t{Tadf::extents{1{t{}1008}}}}}}}}'}  PortWindowSizes={0.000000000000000000e+00; 1.008000000000000000e+03}  PortWindowMargins={0.000000000000000000e+00; 0.000000000000000000e+00}  PortSynchronicities={'auto', 'sync'}  PortSignalSizes={0.000000000000000000e+00; 0.000000000000000000e+00}  ClassTemplateSpecKind=none  ClassTemplateParamNames={}  ClassTemplateParamKinds={}  ClassTemplateParamTypes={}  ClassTemplateParamValues={}  ClassCtorParamNames={}  ClassCtorParamSerializedTypes={}  ClassCtorParamValues={}  ClassIndex=1  ClassCtorIndex=0  ClassTabVisible=on  ClassTemplateParamsVisible=off  ClassCtorDeclVisible=off  ClassCtorParamsVisible=off  FunctionTabVisible=on  FunctionDecl=|  PortAttrs={ 'input', 'acc_i', 'input_cascade< cacc64, void > * restrict', '', '', '', ''; 'output', 'sig_o', 'adf::output_buffer< cint16, adf::extents< 1008 > > & restrict', '1008', '', 'sync', '' }  PortAttrsEnables={'off', 'off', 'off', 'off', 'off', 'off', 'off';'off', 'off', 'off', 'off', 'off', 'off', 'off'}  SampleTime=-1  ClassDeclTypeOptions=C[1 1]@t13@class dft7_2;  ClassDecl=class dft7_2;  ClassTemplateParams={}  ClassTemplateParamsEnables={}  ClassCtorDeclTypeOptions=C[1 1]@t7@<empty>  ClassCtorDecl=<empty>  ClassCtorParams={}  KernelHeaderFile=dft7_mmul2.h  KernelClassName=dft7_2  KernelFunction=run  KernelSourceFile=dft7_mmul2.cpp  KernelSearchPaths={'./aie/dft7'}  PreProcOptions={}  blockJsonConstraints="{\"type\":\"constraint\",\"constraintType\":\"location_kernel\",\"sid\":\"36\",\"lhs\":{\"type\":\"location\",\"templParam\":\"kernel\",\"args\":{\"type\":\"kernel\",\"name\":\"pfa1008/pfa1008_dut/pfa1008_aie/dft7/mmul2\",\"sid\":\"36\"}},\"rhs\":{\"type\":\"tile\",\"args\":[{\"type\":\"evaluable\",\"expr\":\"20\",\"value\":20},{\"type\":\"evaluable\",\"expr\":\"0\",\"value\":0}]},\"equality\":true}"
      KernelAllAttrs=|
      | s[12;12;9;9;19;14;21;23;21;23;24;21;15;17;12;24;26;26;26;27;28;9;21;23;23;23;24;25;14;19;19;29]@FunctionNameDeclFileNamePortNamesPortTypesPortSerializedTypesPortDirectionsPortWindowSizeEnablesPortWindowMarginEnablesPortBufferSizeEnablesPortBufferMarginEnablesPortSynchronicityEnablesPortSignalSizeEnablesPortBufferSizesPortBufferMarginsFunctionDeclFunctionTemplateSpecKindFunctionTemplateParamNamesFunctionTemplateParamKindsFunctionTemplateParamTypesFunctionTemplateParamValuesFunctionTemplateParamEnablesClassDeclClassTemplateSpecKindClassTemplateParamNamesClassTemplateParamKindsClassTemplateParamTypesClassTemplateParamValuesClassTemplateParamEnablesClassCtorDeclsClassCtorParamNamesClassCtorParamTypesClassCtorParamSerializedTypes[1 1]@C[32 1]@t3@runt26@../../../dft7/dft7_mmul2.hC[2 1]@t5@acc_it5@sig_oC[2 1]@t40@input_cascade< cacc64, void > * restrictt61@adf::output_buffer< cint16, adf::extents< 1008 > > & restrictC[2 1]@t45@{Q2{P{Tinput_cascade{2{t{Scacc64}}{t{Bv}}}}}}t73@{Q2{R{Tadf::output_buffer{2{t{Scint16}}{t{Tadf::extents{1{t{}1008}}}}}}}}C[2 1]@t5@inputt6@outputC[2 1]@l0@l1@C[2 1]@l0@l0@C[2 1]@l0@l1@C[2 1]@l0@l0@C[2 1]@l0@l1@C[2 1]@l0@l0@C[2 1]@nt4@1008C[2 1]@nnt134@void dft7_2::
      | run(input_cascade< cacc64, void > * restrict acc_i, adf::output_buffer< cint16, adf::extents< 1008 > > & restrict sig_o)t4@nonee[0 1]@e[0 1]@e[0 1]@e[0 1]@e[0 1]@t13@class dft7_2;t4@nonee[0 1]@e[0 1]@e[0 1]@e[0 1]@e[0 1]@e[0 1]@e[0 1]@e[0 1]@e[0 1]@
      FunctionDecl=|
      | void dft7_2::
      | run(input_cascade< cacc64, void > * restrict acc_i, adf::output_buffer< cint16, adf::extents< 1008 > > & restrict sig_o)
  Out1 : Outport
  wires:
  FIFO/1 -> mmul1/2
  FIFO1/1 -> mmul0/1
  mmul0/1 -> mmul1/1
  In1/1 -> FIFO/1, FIFO1/1
  mmul1/1 -> mmul2/1
  mmul2/1 -> Out1/1
